simulink model "Homework2"  (R2017b)
settings: Solver=ode45  StartTime=0.0  StopTime=127  FixedStep=0.1  RelTol=1e-3  EnableMultiTasking=on
PreLoadFcn:
  | RTWConfigurationCB('preloadfcn', bdroot);
InitFcn:
  | parameterVehicle
StopFcn:
  | myAnimation(xActEst,yActEst,thetaAct,X_array,Y_array,rp1,rp2)
  | myStopFcn2sim(xActEst,yActEst,X_array,Y_array,rp1,rp2)
values from neighbouring files (symbols this model uses):
  b = 0.5842    [parameterVehicle.m]
  dcArray = [-100  -30 0  30  100]    [parameterVehicle.m]
  rl = 1*rNominal    (= 0.052959)    [parameterVehicle.m]
  rr = 1*rNominal    (= 0.052959)    [parameterVehicle.m]
  thetaIC = 0*(pi/180)    (= 0)    [parameterVehicle.m]
  wArray = [-Vmax, 0, 0,  0, Vmax]./rNominal    [parameterVehicle.m]
  xIC = 0    [parameterVehicle.m]
  yIC = 0    [parameterVehicle.m]
CloseFcn:
  | rtwprivate ssgencode ModelCloseRequest track_vehicle6_v2
settings Model: Creator=Dogan  LastModifiedBy=soutrik
settings DataIOCC: LimitDataPoints=on  SaveFormat=Array  SignalLoggingSaveFormat=ModelDataLogs
settings OptimizationCC: ExpressionDepthLimit=2147483647  InitFltsAndDblsToZero=on  LifeSpan=inf
settings DebuggingCC: SaveWithParameterizedLinksMsg=none  UnderspecifiedInitializationDetection=Classic  MergeDetectMultiDrivingBlocksExec=none  SignalResolutionControl=TryResolveAllWithWarning  SolverPrmCheckMsg=warning  MultiTaskDSMMsg=warning  MultiTaskCondExecSysMsg=none  FcnCallInpInsideContextMsg=warning  StateNameClashWarn=warning  SFUnexpectedBacktrackingDiag=warning  SFNoUnconditionalDefaultTransitionDiag=warning  SFExecutionAtInitializationDiag=none
settings HardwareCC: ProdBitPerLong=64  ProdLargestAtomicFloat=None  ProdHWDeviceType=Intel->x86-64  TargetHWDeviceType=32-bit Generic
settings ModelReferenceCC: PropagateSignalLabelsOutOfModel=off
settings SFSimCC: SimParseCustomCode=off
settings RTWCC: Description=Generic Real-Time Target
settings CodeAppCC: GenerateComments=off  SimulinkBlockComments=off
settings GRTTargetCC: TargetLangStandard=C89/C90 (ANSI)  GeneratePreprocessorConditionals=Disable all
settings ConfigComp: CovMetricSettings=dw  CovHtmlReporting=on  CovSaveCumulativeToWorkspaceVar=on  CovSaveSingleToWorkspaceVar=on  CovExternalEMLEnable=off

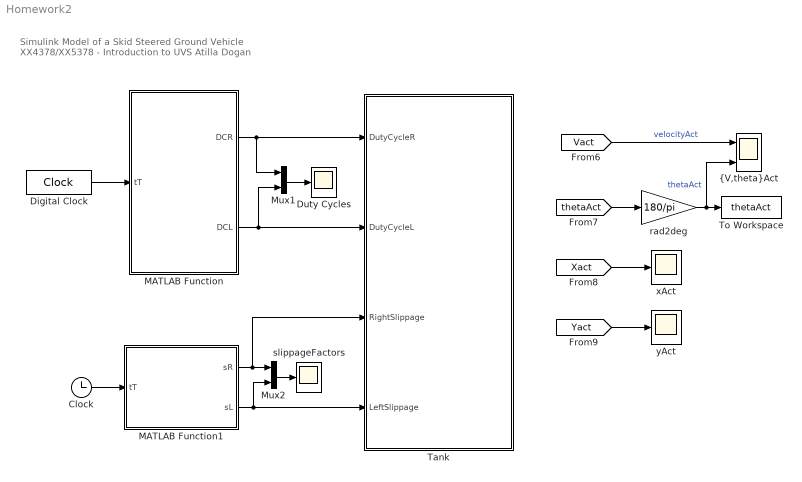
== system Homework2 ==
  note: Simulink Model of a Skid Steered Ground Vehicle
      | XX4378/XX5378 - Introduction to UVS
      | Atilla Dogan
  Clock : Clock
  Digital Clock : DigitalClock  SampleTime=.1
  Duty Cycles : Scope
  MATLAB Function : MATLAB Function  TreatAsAtomicUnit=on
  MATLAB Function1 : MATLAB Function  TreatAsAtomicUnit=on
  Mux1 : Mux  Inputs=2
  Mux2 : Mux  Inputs=2
  Tank : Subsystem
  To Workspace : ToWorkspace  VariableName=thetaAct  SaveFormat=Structure With Time  SampleTime=-1
  rad2deg : Gain  Gain=180/pi
  slippageFactors : Scope
  xAct : Scope
  yAct : Scope
  "{V,theta}Act" : Scope  NumInputPorts=2
  wires:
  rad2deg/1 -> "{V,theta}Act"/2, To Workspace/1  "thetaAct"
  MATLAB Function1/1(sR) -> Tank/3(RightSlippage), Mux2/1
  MATLAB Function1/2(sL) -> Tank/4(LeftSlippage), Mux2/2
  Clock/1 -> MATLAB Function1/1(tT)
  [Vact] -> "{V,theta}Act"/1  "velocityAct"
  [thetaAct] -> rad2deg/1
  [Xact] -> xAct/1
  [Yact] -> yAct/1
  MATLAB Function/1(DCR) -> Mux1/1, Tank/1(DutyCycleR)
  MATLAB Function/2(DCL) -> Mux1/2, Tank/2(DutyCycleL)
  Digital Clock/1 -> MATLAB Function/1(tT)
  Mux2/1 -> slippageFactors/1
  Mux1/1 -> Duty Cycles/1

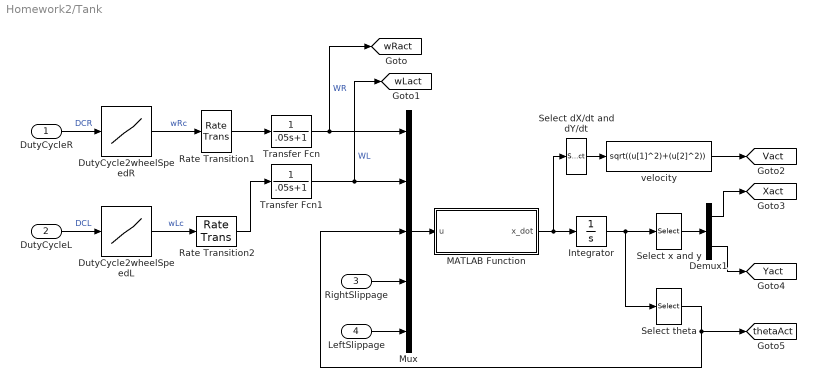
== system Homework2/Tank ==
  DutyCycleR : Inport
  DutyCycleL : Inport  Port=2
  RightSlippage : Inport  Port=3
  LeftSlippage : Inport  Port=4
  Demux1 : Demux  Outputs=2
  DutyCycle2wheelSpeedL : Lookup  InputValues=dcArray  Table=wArray  LookUpMeth=Interpolation-Use End Values
  DutyCycle2wheelSpeedR : Lookup  InputValues=dcArray  Table=wArray  LookUpMeth=Interpolation-Use End Values
  Integrator : Integrator  InitialCondition=[xIC; yIC ; thetaIC]
  MATLAB Function : MATLAB Function  TreatAsAtomicUnit=on
  Mux : Mux  Inputs=5
  Rate Transition1 : RateTransition
  Rate Transition2 : RateTransition
  Select dX/dt and dY/dt : Selector  InputPortWidth=3  IndexOptions=Index vector (dialog)  Indices=[1 2]  OutputSizes=1
  Select theta : Selector  InputPortWidth=3  IndexOptions=Index vector (dialog)  Indices=3  OutputSizes=1
  Select x and y : Selector  InputPortWidth=3  IndexOptions=Index vector (dialog)  Indices=[1 2]  OutputSizes=1
  Transfer Fcn : TransferFcn  Denominator=[.05 1]
  Transfer Fcn1 : TransferFcn  Denominator=[.05 1]
  velocity : Fcn  Expr=sqrt((u[1]^2)+(u[2]^2))
  tag scope: Vact=global, Xact=global, Yact=global, thetaAct=global, wLact=global, wRact=global
  wires:
  DutyCycleL/1 -> DutyCycle2wheelSpeedL/1  "DCL"
  DutyCycleR/1 -> DutyCycle2wheelSpeedR/1  "DCR"
  DutyCycle2wheelSpeedL/1 -> Rate Transition2/1  "wLc"
  DutyCycle2wheelSpeedR/1 -> Rate Transition1/1  "wRc"
  Rate Transition2/1 -> Transfer Fcn1/1
  Rate Transition1/1 -> Transfer Fcn/1
  Demux1/2 -> [Yact]
  Demux1/1 -> [Xact]
  Select x and y/1 -> Demux1/1
  velocity/1 -> [Vact]
  Select dX/dt and dY/dt/1 -> velocity/1
  MATLAB Function/1(x_dot) -> Integrator/1, Select dX/dt and dY/dt/1
  Select theta/1 -> [thetaAct], Mux/3
  Transfer Fcn1/1 -> [wLact], Mux/2  "WL"
  Transfer Fcn/1 -> [wRact], Mux/1  "WR"
  LeftSlippage/1 -> Mux/5
  RightSlippage/1 -> Mux/4
  Mux/1 -> MATLAB Function/1(u)
  Integrator/1 -> Select theta/1, Select x and y/1

== matlab function Homework2/Tank/MATLAB Function ==
  data: u input; x_dot output; b parameter; rr parameter; rl parameter
function x_dot = fcn(u,b,rr,rl)
%#codegen

wr = u(1);
wl = u(2);
theta = u(3);
sr = u(4);
sl = u(5);
x_dot = [((1-sl)*rl*wl + (1-sr)*rr*wr)*cos(theta)/2;
         ((1-sl)*rl*wl + (1-sr)*rr*wr)*sin(theta)/2;
         ((1-sl)*rl*wl - (1-sr)*rr*wr)/b];

== matlab function Homework2/MATLAB Function ==
  data: tT input; DCR output; DCL output
function [DCR,DCL] = inputDC(tT)
%#codegen

% tT  : time
% DCR: Duty Cycle Right 
% DCL: Duty Cycle Left 

% initialization
DCR=0;DCL=0;

if tT > 10
    DCR=70; 
    DCL=70; 
end

    if tT > 20 && tT < 30
    DCR = 44; 
    DCL = 23;
    end
    
if tT > 45 && tT < 50
    DCR = 14; 
    DCL = 64;
end

if tT > 50 && tT < 54
    DCR = 9;
    DCL = 59.5;
end

if tT > 76 && tT < 80
    DCR = 77;
    DCL = 15;
end

if tT > 90 && tT < 100
    DCR = 17;
    DCL = 61.75;
end

== matlab function Homework2/MATLAB Function1 ==
  data: tT input; sR output; sL output
function [sR,sL] = slipFnc(tT)
%#codegen

% tT  : time
% sR  : slippage on Right Track
% sL  : slippage on Left Track

% initialization
sR=0;sL=0;

% 
% if tT > 25
%    sR=0;
%    sL=0.2;
% end
  

% if tT > 20 && tT < 25
% %     sR=0.2;
%     sL=0.2;
% end
%
